simulink model "TestDiscreteTime"  (R2022a)
settings: Solver=VariableStepAuto  StartTime=0.0  StopTime=t_final  RelTol=1e-3
values from neighbouring files (symbols this model uses):
  A = [-(1/SIM.R_1+1/SIM.R_2)  1/SIM.R_2             0 ... (first row only)    [DAE_Circuit_main.m]    (also in TestDiscreteTimeSimulink.m = 1e-3*eye(2))
  A_DT = SS_DT.A    [TestDiscreteTimeSimulink.m]
  B = [1/SIM.R_1 ; 0 ; 0]    [DAE_Circuit_main.m]    (also in TestDiscreteTimeSimulink.m = 1*ones(2,1))
  B_DT = SS_DT.B    [TestDiscreteTimeSimulink.m]
  C = [0 0 1]    [DAE_Circuit_main.m]    (also in SimulinkInput.mat = [1  0  0; 0  1  0; 0  0  1]; Test.mat = [1 0 0]; TestDiscreteTimeSimulink.m = [1 0)
  multiple = 100    [TestDiscreteTimeSimulink.m]
  Ts_sample = 1    [TestDiscreteTimeSimulink.m]
settings Model: Creator=tyevans  LastModifiedBy=tyevans

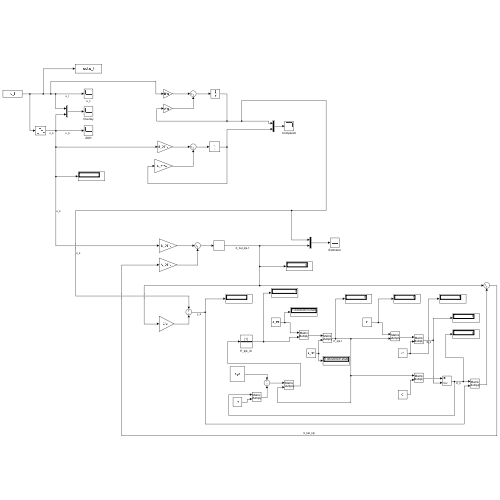
[thumbnail: Simulink's stored preview of the top-level diagram]
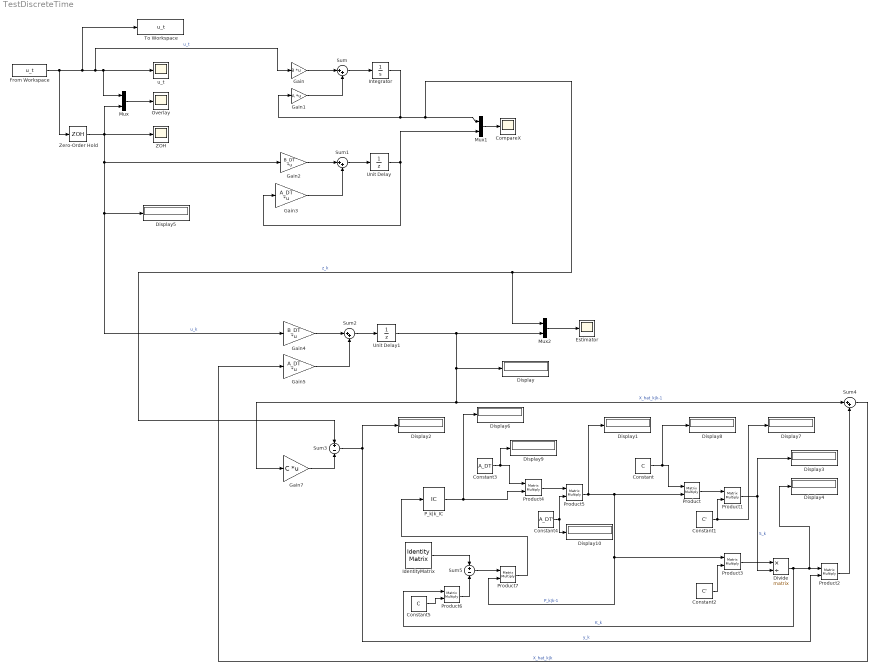
== system TestDiscreteTime ==
  CompareX : Scope
  Constant : Constant  Value=C  VectorParams1D=off
  Constant1 : Constant  Value=C'  VectorParams1D=off
  Constant2 : Constant  Value=C'  VectorParams1D=off
  Constant3 : Constant  Value=A_DT  VectorParams1D=off
  Constant4 : Constant  Value=A_DT'  VectorParams1D=off
  Constant5 : Constant  Value=C  VectorParams1D=off
  Display{,1..10} (11 alike) : Display
      Display10 settings: Decimation=5
      Display9 settings: Decimation=5
  Divide : Product  Inputs=*/  Multiplication=Matrix(*)
  Estimator : Scope
  From Workspace : FromWorkspace  VariableName=u_t  SampleTime=Ts_sample/multiple  OutputAfterFinalValue=Holding final value
  Gain : Gain  Gain=B  Multiplication=Matrix(K*u)
  Gain1 : Gain  Gain=A  Multiplication=Matrix(K*u)
  Gain2 : Gain  Gain=B_DT  Multiplication=Matrix(K*u)
  Gain3 : Gain  Gain=A_DT  Multiplication=Matrix(K*u)
  Gain4 : Gain  Gain=B_DT  Multiplication=Matrix(K*u)
  Gain5 : Gain  Gain=A_DT  Multiplication=Matrix(K*u)
  Gain7 : Gain  Gain=C  Multiplication=Matrix(K*u)
  IdentityMatrix : IdentityMatrix  OutputDimensions=1  SampleTime=Ts_sample
  Integrator : Integrator
  Mux : Mux  Inputs=2
  Mux1 : Mux  Inputs=2
  Mux2 : Mux  Inputs=2
  Overlay : Scope
  P_k|k_IC : InitialCondition
  Product{,1..7} (8 alike) : Product  Multiplication=Matrix(*)
  Sum{,1..2,4} (4 alike) : Sum  Inputs=|++
  Sum3 : Sum  Inputs=+-
  Sum5 : Sum  Inputs=+-
  To Workspace : ToWorkspace  VariableName=u_t  SaveFormat=Timeseries  SampleTime=-1
  Unit Delay : UnitDelay  SampleTime=-1  HasFrameUpgradeWarning=on
  Unit Delay1 : UnitDelay  SampleTime=-1  HasFrameUpgradeWarning=on
  ZOH : Scope
  Zero-Order Hold : ZeroOrderHold  SampleTime=Ts_sample
  u_t : Scope
  wires:
  From Workspace/1 -> Zero-Order Hold/1, To Workspace/1, Gain/1, Mux/1, u_t/1  "u_t"
  Mux/1 -> Overlay/1
  Gain/1 -> Sum/1
  Gain1/1 -> Sum/2
  Sum/1 -> Integrator/1
  Gain3/1 -> Sum1/2
  Unit Delay/1 -> Gain3/1, Mux1/2
  Sum1/1 -> Unit Delay/1
  Gain2/1 -> Sum1/1
  Mux1/1 -> CompareX/1
  Sum2/1 -> Unit Delay1/1
  Gain4/1 -> Sum2/1
  Gain5/1 -> Sum2/2
  Zero-Order Hold/1 -> Display5/1, Gain4/1, Gain2/1, Mux/2, ZOH/1  "u_k"
  Unit Delay1/1 -> Display/1, Gain7/1, Sum4/1, Mux2/2  "X_hat_k|k-1"
  Gain7/1 -> Sum3/2
  Integrator/1 -> Mux1/1, Sum3/1, Mux2/1, Gain1/1  "z_k"
  Sum3/1 -> Product2/2, Display2/1  "y_k"
  Constant/1 -> Display8/1, Product/1
  Product/1 -> Product1/1
  Constant1/1 -> Product1/2, Display7/1
  Product1/1 -> Display3/1, Divide/2  "S_k"
  Constant2/1 -> Product3/2
  Product3/1 -> Divide/1
  Constant3/1 -> Display9/1, Product4/1
  Product7/1 -> P_k|k_IC/1
  Product4/1 -> Product5/1
  Constant4/1 -> Product5/2, Display10/1
  Product5/1 -> Display1/1, Product7/2, Product3/1, Product/2  "P_k|k-1"
  Divide/1 -> Product6/1, Display4/1, Product2/1  "K_k"
  Product2/1 -> Sum4/2
  Sum4/1 -> Gain5/1  "X_hat_k|k"
  IdentityMatrix/1 -> Sum5/1
  Product6/1 -> Sum5/2
  Constant5/1 -> Product6/2
  Sum5/1 -> Product7/1
  Mux2/1 -> Estimator/1
  P_k|k_IC/1 -> Display6/1, Product4/2
